simulink model "controllore_stato_integrale_new"  (R2014b)
settings: Solver=ode45  SolverMode=SingleTasking  StartTime=0.0  StopTime=simulation_time  RelTol=1e-3
values from neighbouring files (symbols this model uses):
  A = [0, 1 ... (first row only)    [controllo_motore_modello_interno.m]    (also in controllo_motore_stato.m; controllo_motore_stato_integrale.m)
  B = [0 ... (first row only)    [controllo_motore_modello_interno.m]    (also in controllo_motore_stato.m; controllo_motore_stato_integrale.m)
  C = [c, 0]    [controllo_motore_modello_interno.m]    (also in controllo_motore_stato.m = [ c , 0]; controllo_motore_stato_integrale.m)
  d = 0    [controllo_motore_stato.m]    (also in controllo_motore_stato_integrale.m = -0.2; modello_motore.m = -0.5)
  K = acker (Az , Bz , W)    [controllo_motore_modello_interno.m]    (also in controllo_motore_stato.m = place ( A , B , W ); controllo_motore_stato_integrale.m = acker (Az, Bz, W))
  Kg2v = 5 / 176    (= 0.0284090909091)    [controllo_motore_modello_interno.m]    (also in controllo_motore_stato.m; controllo_motore_stato_integrale.m; modello_motore.m)
  Ki = K(1)    [controllo_motore_stato_integrale.m]
  r = 50    [controllo_motore_stato.m]    (also in controllo_motore_stato_integrale.m = 120; modello_motore.m = 120)
  step_time_input = 1    [controllo_motore_modello_interno.m]    (also in controllo_motore_stato.m; controllo_motore_stato_integrale.m; modello_motore.m)
settings Model: Creator=User  LastModifiedBy=Nicola
settings DataIOCC: SignalLoggingSaveFormat=ModelDataLogs
settings OptimizationCC: BlockReduction=off  BooleanDataType=off
settings DebuggingCC: SaveWithParameterizedLinksMsg=none  UnderspecifiedInitializationDetection=Classic  MergeDetectMultiDrivingBlocksExec=none  SignalResolutionControl=TryResolveAllWithWarning  SolverPrmCheckMsg=none  MultiTaskDSMMsg=warning  MultiTaskCondExecSysMsg=none  StateNameClashWarn=warning
settings HardwareCC: TargetUnknown=on
settings RTWCC: IncludeERTFirstTime=on

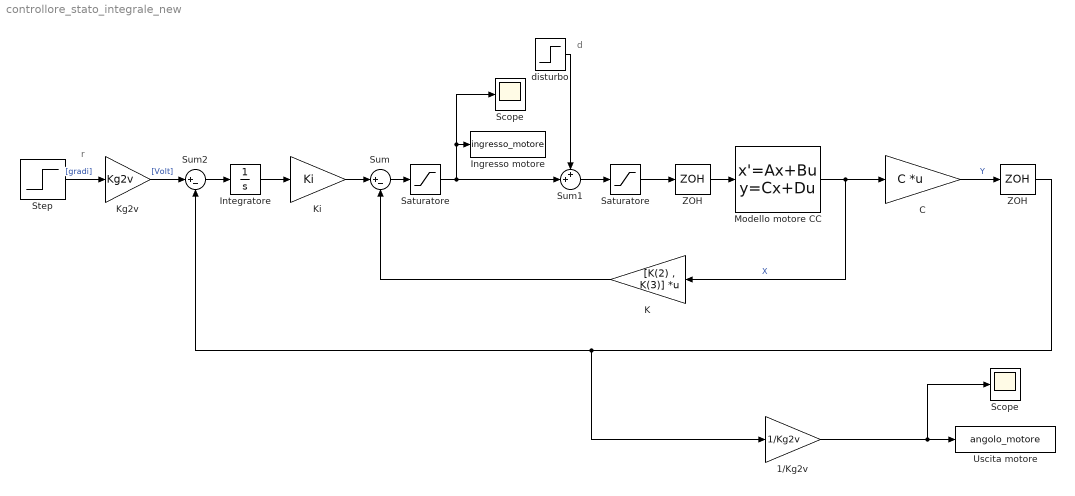
== system controllore_stato_integrale_new ==
  note: d
  note: r
  "1/Kg2v " : Gain  Gain=1/Kg2v
  C : Gain  Gain=C  Multiplication=Matrix(K*u) (u vector)
  Ingresso motore : ToWorkspace  VariableName=ingresso_motore  SampleTime=-1
  Integratore : Integrator
  K : Gain  Gain=[K(2) , K(3)]  Multiplication=Matrix(K*u) (u vector)
  Kg2v : Gain  Gain=Kg2v
  Ki : Gain  Gain=Ki
  Modello motore CC : StateSpace  A=A  B=B  C=[1 , 0 ; 0 , 1]  D=[0 ; 0]  X0=0
  Saturatore : Saturate  UpperLimit=5  LowerLimit=-5
  "Saturatore " : Saturate  UpperLimit=5  LowerLimit=-5
  Scope : Scope
  "Scope " : Scope
  Step : Step  Time=step_time_input  After=r  SampleTime=0
  Sum : Sum  Inputs=|+-
  Sum1 : Sum  Inputs=++|
  Sum2 : Sum  Inputs=|+-
  Uscita motore : ToWorkspace  VariableName=angolo_motore  SampleTime=-1
  ZOH : ZeroOrderHold  SampleTime=0.001
  "ZOH " : ZeroOrderHold  SampleTime=0.001
  disturbo : Step  Time=step_time_input  After=d  SampleTime=0
  wires:
  Modello motore CC/1 -> C/1, K/1  "X"
  Saturatore/1 -> ZOH/1
  ZOH/1 -> Modello motore CC/1
  C/1 -> "ZOH "/1  "Y"
  Sum/1 -> "Saturatore "/1
  Step/1 -> Kg2v/1  "[gradi]"
  "Saturatore "/1 -> Sum1/2, Ingresso motore/1, "Scope "/1
  "1/Kg2v "/1 -> Scope/1, Uscita motore/1
  K/1 -> Sum/2
  Ki/1 -> Sum/1
  Integratore/1 -> Ki/1
  Sum2/1 -> Integratore/1
  "ZOH "/1 -> "1/Kg2v "/1, Sum2/2
  disturbo/1 -> Sum1/1
  Sum1/1 -> Saturatore/1
  Kg2v/1 -> Sum2/1  "[Volt]"
